simulink model "Simulacion"  (R2021a)
settings: Solver=VariableStepAuto  StartTime=0.0  StopTime=10.0  RelTol=1e-3
values from neighbouring files (symbols this model uses):
  ue = 1/2    (= 0.5)    [Compensacion.m]    (also in Linealizacion.m = 0)
  x1e = pi/6    (= 0.523598775598)    [Compensacion.m]    (also in Linealizacion.m = 0)
  x2e = 0    [Compensacion.m]    (also in Linealizacion.m = 0.785398163397)
  ye = pi/6    (= 0.523598775598)    [Compensacion.m]    (also in Linealizacion.m = 0.785398163397)
libraries: cstblocks x5
settings Model: Creator=Santiago  LastModifiedBy=Santiago

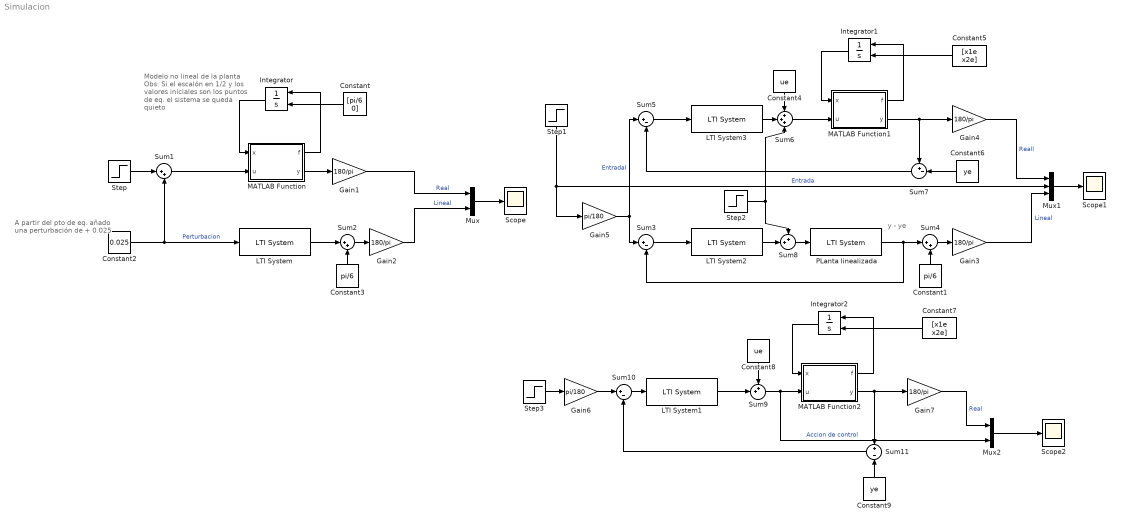
== system Simulacion ==
  note: y - ye
  note: A partir del pto de eq. añado una perturbación
      | de + 0.025
  note: Modelo no lineal de la planta
      | Obs: Si el escalón en 1/2
      | y los valores iniciales
      | son los puntos de eq. el
      | sistema se queda quieto
  Constant : Constant  Value=[pi/6 0]
  Constant1 : Constant  Value=pi/6
  Constant2 : Constant  Value=0.025
  Constant3 : Constant  Value=pi/6
  Constant4 : Constant  Value=ue
  Constant5 : Constant  Value=[x1e x2e]
  Constant6 : Constant  Value=ye
  Constant7 : Constant  Value=[x1e x2e]
  Constant8 : Constant  Value=ue
  Constant9 : Constant  Value=ye
  Gain{1..4,7} (5 alike) : Gain  Gain=180/pi
  Gain5 : Gain  Gain=pi/180
  Gain6 : Gain  Gain=pi/180
  Integrator : Integrator  InitialConditionSource=external
  Integrator1 : Integrator  InitialConditionSource=external
  Integrator2 : Integrator  InitialConditionSource=external
  LTI System : cstblocks/LTI System  sys=P  IC=[]
  LTI System1 : cstblocks/LTI System  sys=C_digi  IC=[]
  LTI System2 : cstblocks/LTI System  sys=C  IC=[]
  LTI System3 : cstblocks/LTI System  sys=C  IC=[]
  MATLAB Function : MATLAB Function  TreatAsAtomicUnit=on
  MATLAB Function1 : MATLAB Function  TreatAsAtomicUnit=on
  MATLAB Function2 : MATLAB Function  TreatAsAtomicUnit=on
  Mux : Mux  Inputs=2
  Mux1 : Mux  Inputs=3
  Mux2 : Mux  Inputs=2
  PLanta linealizada : cstblocks/LTI System  sys=P  IC=[]
  Scope : Scope
  Scope1 : Scope
  Scope2 : Scope
  Step : Step  Time=0  After=1/2  SampleTime=0
  Step1 : Step  After=5  SampleTime=0
  Step2 : Step  Time=5  After=0.5  SampleTime=0
  Step3 : Step  After=5  SampleTime=0
  Sum1 : Sum  Inputs=|++
  Sum10 : Sum  Inputs=|+-
  Sum11 : Sum  Inputs=+|-
  Sum2 : Sum  Inputs=|++
  Sum3 : Sum  Inputs=|+-
  Sum4 : Sum  Inputs=|++
  Sum5 : Sum  Inputs=|+-
  Sum6 : Sum  Inputs=+++
  Sum7 : Sum  Inputs=+-|
  Sum8 : Sum  Inputs=++|
  Sum9 : Sum  Inputs=++|
  wires:
  MATLAB Function/1(f) -> Integrator/1
  Integrator/1 -> MATLAB Function/1(x)
  Constant/1 -> Integrator/2
  Constant2/1 -> LTI System/1, Sum1/2  "Perturbacion"
  Step/1 -> Sum1/1
  Sum1/1 -> MATLAB Function/2(u)
  LTI System/1 -> Sum2/1
  Constant3/1 -> Sum2/2
  Mux/1 -> Scope/1
  MATLAB Function/2(y) -> Gain1/1
  Sum2/1 -> Gain2/1
  Gain1/1 -> Mux/1  "Real"
  Gain2/1 -> Mux/2  "Lineal"
  Sum3/1 -> LTI System2/1
  Mux1/1 -> Scope1/1
  PLanta linealizada/1 -> Sum4/1, Sum3/2
  Constant1/1 -> Sum4/2
  Sum4/1 -> Gain3/1
  Gain3/1 -> Mux1/3  "Lineal"
  Sum6/1 -> MATLAB Function1/2(u)
  Constant5/1 -> Integrator1/2
  MATLAB Function1/1(f) -> Integrator1/1
  Integrator1/1 -> MATLAB Function1/1(x)
  Sum5/1 -> LTI System3/1
  Constant6/1 -> Sum7/2
  Sum7/1 -> Sum5/2
  MATLAB Function1/2(y) -> Gain4/1, Sum7/1
  Gain4/1 -> Mux1/1  "Reall"
  Step1/1 -> Mux1/2, Gain5/1  "Entrada"
  Gain5/1 -> Sum5/1, Sum3/1  "Entradal"
  LTI System3/1 -> Sum6/2
  Constant4/1 -> Sum6/1
  LTI System2/1 -> Sum8/2
  Sum8/1 -> PLanta linealizada/1
  Step2/1 -> Sum8/1, Sum6/3
  Step3/1 -> Gain6/1
  Constant7/1 -> Integrator2/2
  MATLAB Function2/1(f) -> Integrator2/1
  Integrator2/1 -> MATLAB Function2/1(x)
  LTI System1/1 -> Sum9/2
  Sum9/1 -> Mux2/2, MATLAB Function2/2(u)  "Accion de control"
  Constant8/1 -> Sum9/1
  Gain6/1 -> Sum10/1
  Sum10/1 -> LTI System1/1
  Constant9/1 -> Sum11/2
  Sum11/1 -> Sum10/2
  MATLAB Function2/2(y) -> Gain7/1, Sum11/1
  Mux2/1 -> Scope2/1
  Gain7/1 -> Mux2/1  "Real"

== matlab function Simulacion/MATLAB Function ==
  data: x input; f output; u input; y output
function [f, y] = fcn(x, u)

f1 = x(2);
f2 = -sin(x(1)) + u;

f = [f1; f2];

y = x(1);

== matlab function Simulacion/MATLAB Function2 ==
  data: x input; f output; u input; y output
function [f, y] = fcn(x, u)

f1 = x(2);
f2 = -sin(x(1)) + u;

f = [f1; f2];

y = x(1);

== matlab function Simulacion/MATLAB Function1 ==
  data: x input; f output; u input; y output
function [f, y] = fcn(x, u)

f1 = x(2);
f2 = -sin(x(1)) + u;

f = [f1; f2];

y = x(1);
